simulink model "ep4_6_2"  (R2018a)
settings: Solver=VariableStepAuto  StartTime=0.0  StopTime=10.0  MaxStep=0.01  RelTol=1e-6
settings Model: Creator=zheny  LastModifiedBy=zheny

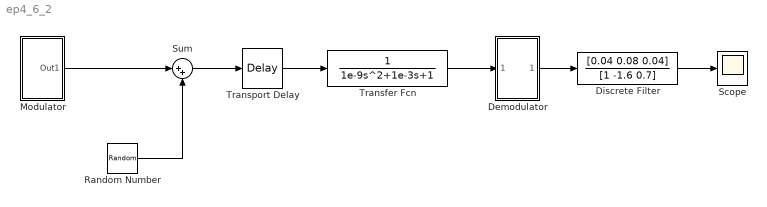
== system ep4_6_2 ==
  Demodulator : Subsystem
  Discrete Filter : DiscreteFilter  Numerator=[0.04 0.08 0.04]  Denominator=[1 -1.6 0.7]  SampleTime=0.005
  Modulator : Subsystem
  Random Number : RandomNumber  Variance=0.01  SampleTime=0.1
  Scope : Scope
  Sum : Sum  Inputs=|++
  Transfer Fcn : TransferFcn  Denominator=[1e-9 1e-3 1]
  Transport Delay : TransportDelay
  wires:
  Sum/1 -> Transport Delay/1
  Transport Delay/1 -> Transfer Fcn/1
  Discrete Filter/1 -> Scope/1
  Random Number/1 -> Sum/2
  Modulator/1(Out1) -> Sum/1
  Transfer Fcn/1 -> Demodulator/1(In1)
  Demodulator/1(Out1) -> Discrete Filter/1

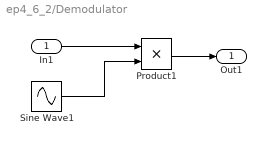
== system ep4_6_2/Demodulator ==
  In1 : Inport
  Product1 : Product
  Sine Wave1 : Sin  Frequency=100  SampleTime=0.005
  Out1 : Outport
  wires:
  Sine Wave1/1 -> Product1/2
  In1/1 -> Product1/1
  Product1/1 -> Out1/1

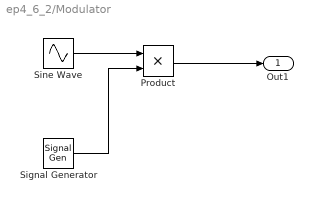
== system ep4_6_2/Modulator ==
  Product : Product
  Signal Generator : SignalGenerator  WaveForm=sawtooth
  Sine Wave : Sin  Frequency=100  SampleTime=0
  Out1 : Outport
  wires:
  Sine Wave/1 -> Product/1
  Signal Generator/1 -> Product/2
  Product/1 -> Out1/1
